simulink model "SimpleYModel"  (R2022a)
settings: Solver=FixedStepAuto  StartTime=0.0  StopTime=10  FixedStep=.01  RelTol=1e-3
settings Model: Creator=hollis  LastModifiedBy=hollis

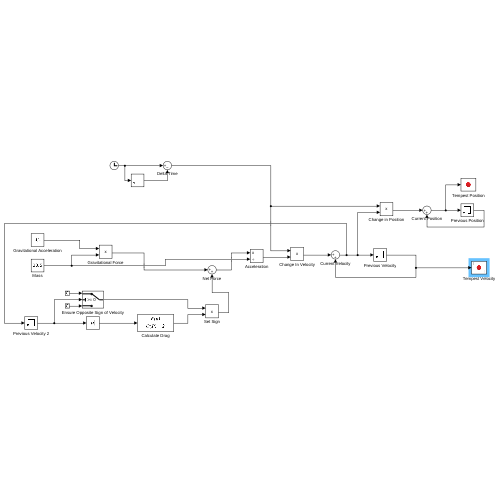
[thumbnail: Simulink's stored preview of the top-level diagram]
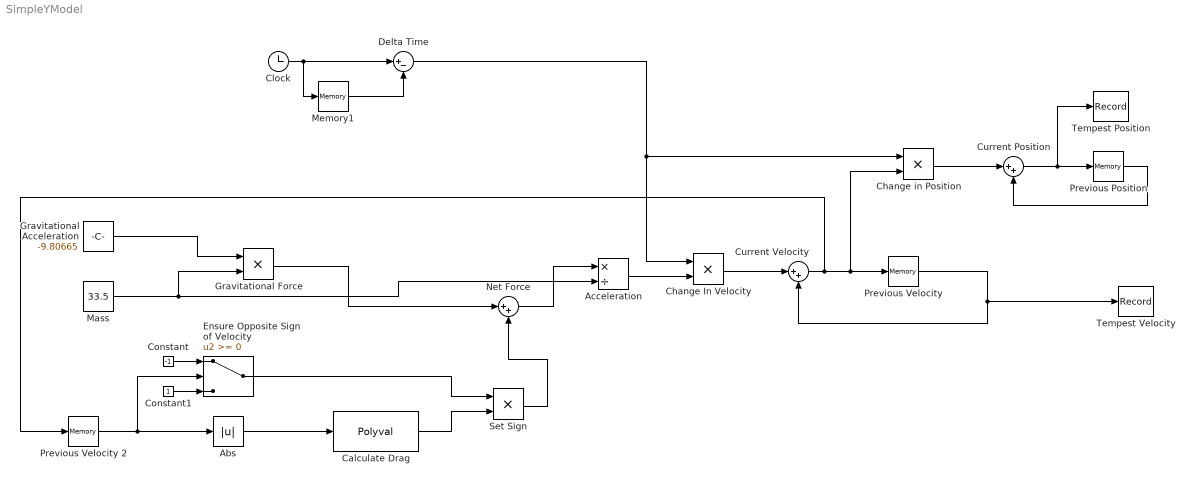
== system SimpleYModel ==
  Abs : Abs  SaturateOnIntegerOverflow=off
  Acceleration : Product  Inputs=*/
  Calculate Drag : Polyval  Coefs=[460, 35, 0]
  Change In Velocity : Product
  Change in Position : Product
  Clock : Clock
  Constant : Constant  Value=-1
  Constant1 : Constant
  Current Position : Sum  Inputs=|++
  Current Velocity : Sum  Inputs=|++
  Delta Time : Sum  Inputs=|+-
  Ensure Opposite Sign of Velocity : Switch  SaturateOnIntegerOverflow=off  InputSameDT=off
  Gravitational Acceleration : Constant  Value=-9.80665
  Gravitational Force : Product
  Mass : Constant  Value=33.5
  Memory1 : Memory
  Net Force : Sum  Inputs=|++
  Previous Position : Memory
  Previous Velocity : Memory
  Previous Velocity 2 : Memory
  Set Sign : Product
  Tempest Position : Record  FileSettingsInternal="{\"entries\":[{\"content\":{\"excelSettings\":{\"content\":{},\"type\":\"Streamout.ExcelSettings\"}},\"type\":\"Streamout.FileSettingStorage\",\"uuid\":\"2a48679f-c499-4075-8ec1-21e073ce2aaf\"}],\"packageUris\":[\"http://schema.mathworks.com/mf0/streamout_blocks/R2020a\"],\"version\":\"1.0\"}"  SignalsInternal="{\"entries\":[{\"content\":{\"signals\":[{\"content\":{\"blockPath\":[\"untitled/Tempest Position\"],\"channel\":[],\"dimensions\":[1],\"domain\":\"untitled/Tempest Position\",\"lineColor\":\"#d95319\",\"plots\":[1],\"port\":1,\"sid\":[\"\"],\"signalID\":6258,\"signalName\":\"Current Position\"},\"type\":\"RecordBlkView.Signal\",\"uuid\":\"e99dbea7-ace3-40c4-92b9-1e6d0ee317bb\"}]},\"type\":\"RecordBlkView.InputSignals\",\"uuid\":\"f4a1a892-fdf6-4545-bf07-c8aaca0fcda9\"}],\"packageUris\":[\"http://schema.mathworks.com/mf0/streamout_blocks/R2020a\"],\"version\":\"1.0\"}"  VisualizationBindings="{\"sparklinesplugin\":{\"info\":[{\"bindingParametersList\":[],\"subplotID\":1}]}}"
  Tempest Velocity : Record  FileSettingsInternal="{\"entries\":[{\"content\":{\"excelSettings\":{\"content\":{},\"type\":\"Streamout.ExcelSettings\"}},\"type\":\"Streamout.FileSettingStorage\",\"uuid\":\"d307a666-5fec-4b90-8581-2db8ba32e067\"}],\"packageUris\":[\"http://schema.mathworks.com/mf0/streamout_blocks/R2020a\"],\"version\":\"1.0\"}"  SignalsInternal="{\"entries\":[{\"content\":{\"signals\":[{\"content\":{\"blockPath\":[\"untitled/Tempest Velocity\"],\"channel\":[],\"dimensions\":[1],\"domain\":\"untitled/Tempest Velocity\",\"lineColor\":\"#edb120\",\"plots\":[1],\"port\":1,\"sid\":[\"\"],\"signalID\":6262,\"signalName\":\"Previous Velocity\"},\"type\":\"RecordBlkView.Signal\",\"uuid\":\"8737cf49-9854-45f1-9691-3b2784e60058\"}]},\"type\":\"RecordBlkView.InputSignals\",\"uuid\":\"c199a170-25e5-49b8-bde0-b0bfce5d9549\"}],\"packageUris\":[\"http://schema.mathworks.com/mf0/streamout_blocks/R2020a\"],\"version\":\"1.0\"}"  VisualizationBindings="{\"sparklinesplugin\":{\"info\":[{\"bindingParametersList\":[],\"subplotID\":1}]}}"
  wires:
  Gravitational Acceleration/1 -> Gravitational Force/1
  Mass/1 -> Acceleration/2, Gravitational Force/2
  Clock/1 -> Memory1/1, Delta Time/1
  Memory1/1 -> Delta Time/2
  Delta Time/1 -> Change In Velocity/1, Change in Position/1
  Change In Velocity/1 -> Current Velocity/1
  Current Velocity/1 -> Previous Velocity 2/1, Change in Position/2, Previous Velocity/1
  Previous Velocity/1 -> Current Velocity/2, Tempest Velocity/1
  Change in Position/1 -> Current Position/1
  Current Position/1 -> Tempest Position/1, Previous Position/1
  Previous Position/1 -> Current Position/2
  Previous Velocity 2/1 -> Abs/1, Ensure Opposite Sign of Velocity/2
  Constant/1 -> Ensure Opposite Sign of Velocity/1
  Constant1/1 -> Ensure Opposite Sign of Velocity/3
  Abs/1 -> Calculate Drag/1
  Calculate Drag/1 -> Set Sign/2
  Ensure Opposite Sign of Velocity/1 -> Set Sign/1
  Acceleration/1 -> Change In Velocity/2
  Set Sign/1 -> Net Force/2
  Gravitational Force/1 -> Net Force/1
  Net Force/1 -> Acceleration/1
